simulink model "SimulinkEcuacionDiferencial"  (R2023b)
settings: Solver=VariableStepAuto  StartTime=0.0  StopTime=10.0  RelTol=1e-6
InitFcn:
  | Parametros
values from neighbouring files (symbols this model uses):
  A = [0 1; -1/P -Q/P]    [Parametros.m]
  B = [0; 1/P]    [Parametros.m]
  C = [1 0]    [Parametros.m]
  D = [0]    [Parametros.m]
  Den = [P Q 1]    [Parametros.m]
  Num = 1    [Parametros.m]
  P = R1*C1*R2*C2    (= 0.223344)    [Parametros.m]
  Q = R1*C2+R2*C2    (= 0.26796)    [Parametros.m]
  U = 5    [Parametros.m]
settings Model: Creator=MiguelFG  LastModifiedBy=MiguelFG

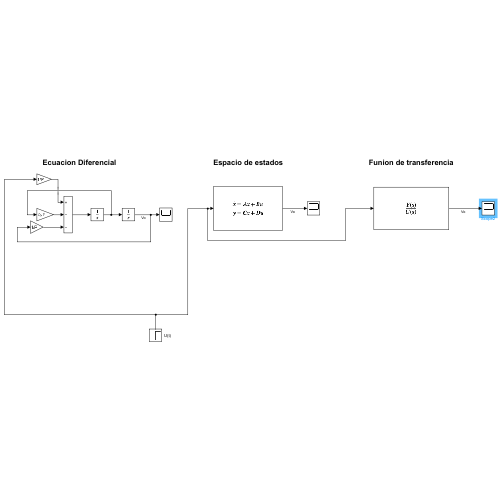
[thumbnail: Simulink's stored preview of the top-level diagram]
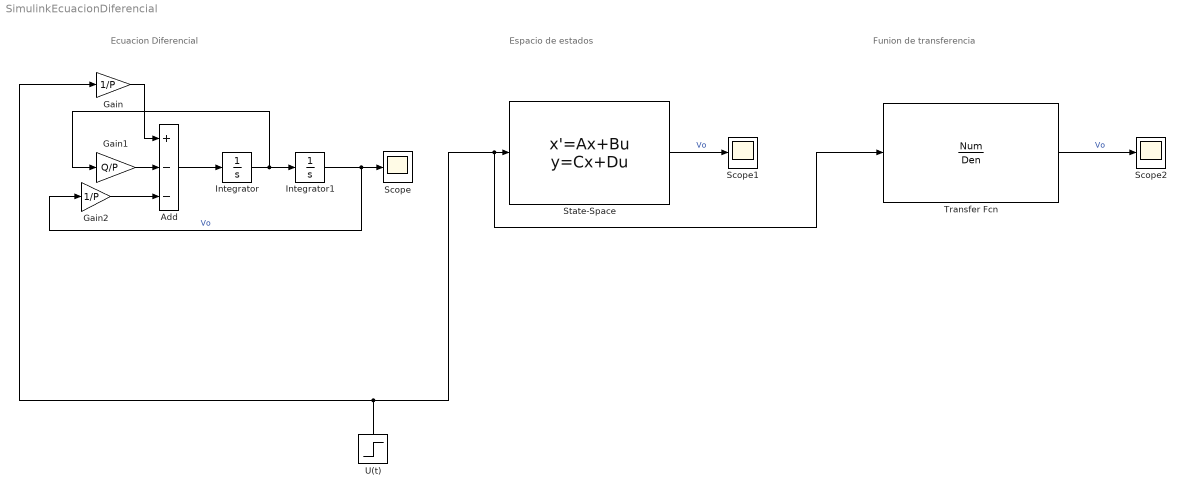
== system SimulinkEcuacionDiferencial ==
  note: Ecuacion Diferencial
  note: Espacio de estados
  note: Funion de transferencia
  Add : Sum  Inputs=+--
  Gain : Gain  Gain=1/P
  Gain1 : Gain  Gain=Q/P
  Gain2 : Gain  Gain=1/P
  Integrator : Integrator
  Integrator1 : Integrator
  Scope : Scope
  Scope1 : Scope
  Scope2 : Scope
  State-Space : StateSpace  A=A  B=B  C=C  D=D  InitialCondition=0
  Transfer Fcn : TransferFcn  Numerator=Num  Denominator=Den
  U(t) : Step  Time=0  After=U  SampleTime=0
  wires:
  Gain2/1 -> Add/3
  Integrator/1 -> Integrator1/1, Gain1/1
  Add/1 -> Integrator/1
  Integrator1/1 -> Gain2/1, Scope/1  "Vo"
  Gain/1 -> Add/1
  Gain1/1 -> Add/2
  State-Space/1 -> Scope1/1  "Vo"
  Transfer Fcn/1 -> Scope2/1  "Vo"
  U(t)/1 -> Gain/1, Transfer Fcn/1, State-Space/1
